simulink model "uavsimblockset_trimModel_Zagi"  (Simulink 8.0)
settings: Solver=ode45  StartTime=0.0  StopTime=10.0  FixedStep=1/30  RelTol=1e-3
undefined symbols (not defined in the file or in its folder): uavsim
libraries: uavsimBlockset_LinearAerodynamicCoefficient x6, uavsimBlockset_LiftCoefficientWithStall x1, aerolibadyn x1, uavsimBlockset_DerivedAerodynamicConditions x1, aerolibtransform2 x1, uavsimBlockset_Environment_calmAtmosphere x1, uavsimBlockset_Quaternion2Rotationvector x1, uavsimblockset_TrimKinematics x1
settings Model: Creator=mstolle  LastModifiedBy=j.bolting
settings DebuggingCC: SolverPrmCheckMsg=none  BusObjectLabelMismatch=error
settings ModelReferenceCC: ModelReferenceMinAlgLoopOccurrences=on

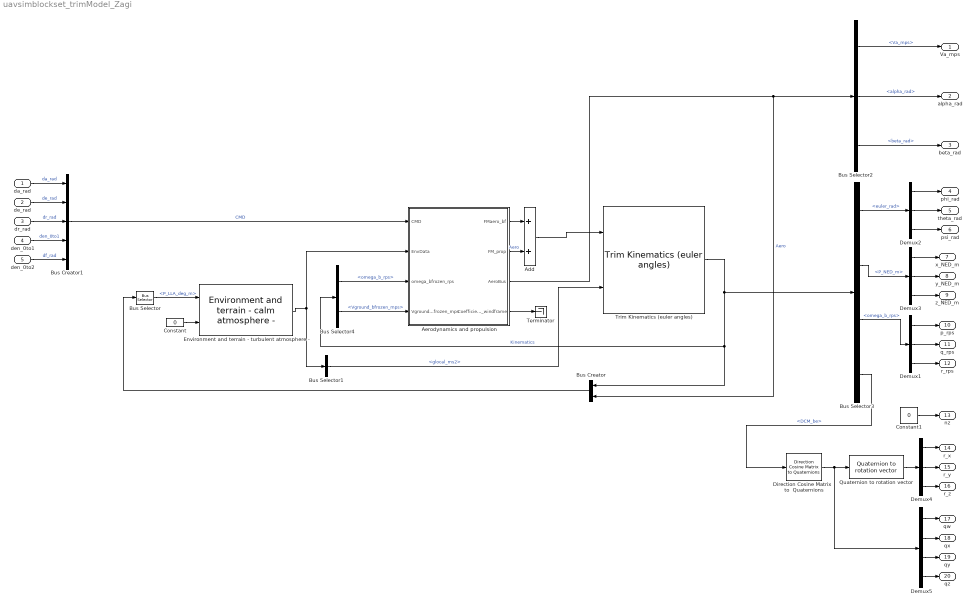
== system uavsimblockset_trimModel_Zagi ==
  da_rad : Inport
  de_rad : Inport  Port=2
  dr_rad : Inport  Port=3
  den_0to1 : Inport  Port=4
  den_0to2 : Inport  Port=5
  Add : Sum
  Aerodynamics and propulsion : Subsystem  AncestorBlock=uavsimBlockset_Zagi_Aerandpropulsion/Zagi aerodynamics and propulsion
      mask Display:
      | port_label('input',1,'CMDBus','texmode','on');
      | port_label('input',2,'EnvDataBus','texmode','on');
      | port_label('input',3,'\omega_{bfrozen,rps}','texmode','on');
      | port_label('input',4,'Vground_{bfrozen,mps}','texmode','on');
      | 
      | port_label('output',1,'FM_{aero}','texmode','on');
      | port_label('output',2,'FM_{propulsion}','texmode','on');
      | port_label('output',3,'AeroBus','texmode','on');
      | port_label('output',4,'C_{wind}','texmode','on');
  Bus Creator1 : BusCreator  Inputs=5  OutDataTypeStr=Bus: CMD  NonVirtualBus=on
  Bus Creator : BusCreator  Inputs=2
  Bus Selector : BusSelector  OutputSignals=Kinematics.Position.P_LLA_deg_m
  Bus Selector1 : BusSelector  OutputSignals=glocal_ms2
  Bus Selector2 : BusSelector  OutputSignals=Va_mps,alpha_rad,beta_rad
  Bus Selector3 : BusSelector  OutputSignals=Attitude.euler_rad,Position.P_NED_m,RotationalVelocity.omega_b_rps,Attitude.DCM_be
  Bus Selector4 : BusSelector  OutputSignals=RotationalVelocity.omega_b_rps,Velocity.Vground_bfrozen_mps
  Constant : Constant  Value=0
  Constant1 : Constant  Value=0
  Demux{1..4} (4 alike) : Demux  Outputs=3
  Demux5 : Demux
  Direction Cosine Matrix   to  Quaternions : aerolibtransform2/Direction Cosine Matrix  to Quaternions
  Environment and terrain - turbulent atmosphere - : uavsimBlockset_Environment_calmAtmosphere/Environment and terrain - calm atmosphere -  SystemSampleTime=-1
  Quaternion to rotation vector : uavsimBlockset_Quaternion2Rotationvector/Quaternion to rotation vector
  Terminator : Terminator
  Trim Kinematics (euler angles) : uavsimblockset_TrimKinematics/Trim Kinematics (euler angles)  mask_inertia=uavsim.zagi.inertiaTensor  mask_mass=uavsim.zagi.mass  mask_P0_ECEF_m=uavsim.mojaveairport_ecef_m  mask_uvw0=[15 0 0]  mask_phithetapsi0=[0 0 0]  mask_omega0=[0 0 0]
  Va_mps : Outport
  alpha_rad : Outport  Port=2
  beta_rad : Outport  Port=3
  phi_rad : Outport  Port=4
  theta_rad : Outport  Port=5
  psi_rad : Outport  Port=6
  x_NED_m : Outport  Port=7
  y_NED_m : Outport  Port=8
  z_NED_m : Outport  Port=9
  p_rps : Outport  Port=10
  q_rps : Outport  Port=11
  r_rps : Outport  Port=12
  nz : Outport  Port=13
  r_x : Outport  Port=14
  r_y : Outport  Port=15
  r_z : Outport  Port=16
  qw : Outport  Port=17
  qx : Outport  Port=18
  qy : Outport  Port=19
  qz : Outport  Port=20
  wires:
  den_0to1/1 -> Bus Creator1/4  "den_0to1"
  de_rad/1 -> Bus Creator1/2  "de_rad"
  da_rad/1 -> Bus Creator1/1  "da_rad"
  dr_rad/1 -> Bus Creator1/3  "dr_rad"
  Bus Creator1/1 -> Aerodynamics and propulsion/1(CMD)  "CMD"
  Environment and terrain - turbulent atmosphere -/1 -> Aerodynamics and propulsion/2(EnvData), Bus Selector1/1
  Bus Selector3/1 -> Demux2/1  "<euler_rad>"
  Demux2/1 -> phi_rad/1
  Demux2/2 -> theta_rad/1
  Demux2/3 -> psi_rad/1
  Bus Selector3/3 -> Demux1/1  "<omega_b_rps>"
  Demux1/1 -> p_rps/1
  Demux1/2 -> q_rps/1
  Demux1/3 -> r_rps/1
  Bus Selector2/1 -> Va_mps/1  "<Va_mps>"
  Bus Selector2/2 -> alpha_rad/1  "<alpha_rad>"
  Bus Selector2/3 -> beta_rad/1  "<beta_rad>"
  Trim Kinematics (euler angles)/1 -> Bus Selector3/1, Bus Creator/1, Bus Selector4/1  "Kinematics"
  Bus Selector4/1 -> Aerodynamics and propulsion/3(omega_bfrozen_rps)  "<omega_b_rps>"
  Bus Selector4/2 -> Aerodynamics and propulsion/4(Vground_bfrozen_mps)  "<Vground_bfrozen_mps>"
  Bus Selector1/1 -> Trim Kinematics (euler angles)/2  "<glocal_ms2>"
  Bus Selector3/2 -> Demux3/1  "<P_NED_m>"
  Demux3/1 -> x_NED_m/1
  Demux3/2 -> y_NED_m/1
  Demux3/3 -> z_NED_m/1
  Constant1/1 -> nz/1
  Bus Selector3/4 -> Direction Cosine Matrix   to  Quaternions/1  "<DCM_be>"
  Direction Cosine Matrix   to  Quaternions/1 -> Demux5/1, Quaternion to rotation vector/1
  Quaternion to rotation vector/1 -> Demux4/1
  Demux4/1 -> r_x/1
  Demux4/2 -> r_y/1
  Demux4/3 -> r_z/1
  Demux5/1 -> qw/1
  Demux5/2 -> qx/1
  Demux5/3 -> qy/1
  Demux5/4 -> qz/1
  den_0to2/1 -> Bus Creator1/5  "df_rad"
  Bus Creator/1 -> Bus Selector/1
  Constant/1 -> Environment and terrain - turbulent atmosphere -/2
  Bus Selector/1 -> Environment and terrain - turbulent atmosphere -/1  "<P_LLA_deg_m>"
  Aerodynamics and propulsion/4(Coefficients_windframe) -> Terminator/1
  Aerodynamics and propulsion/1(FMaero_bf) -> Add/1
  Aerodynamics and propulsion/2(FM_prop) -> Add/2  "Aero"
  Add/1 -> Trim Kinematics (euler angles)/1
  Aerodynamics and propulsion/3(AeroBus) -> Bus Creator/2, Bus Selector2/1  "Aero"

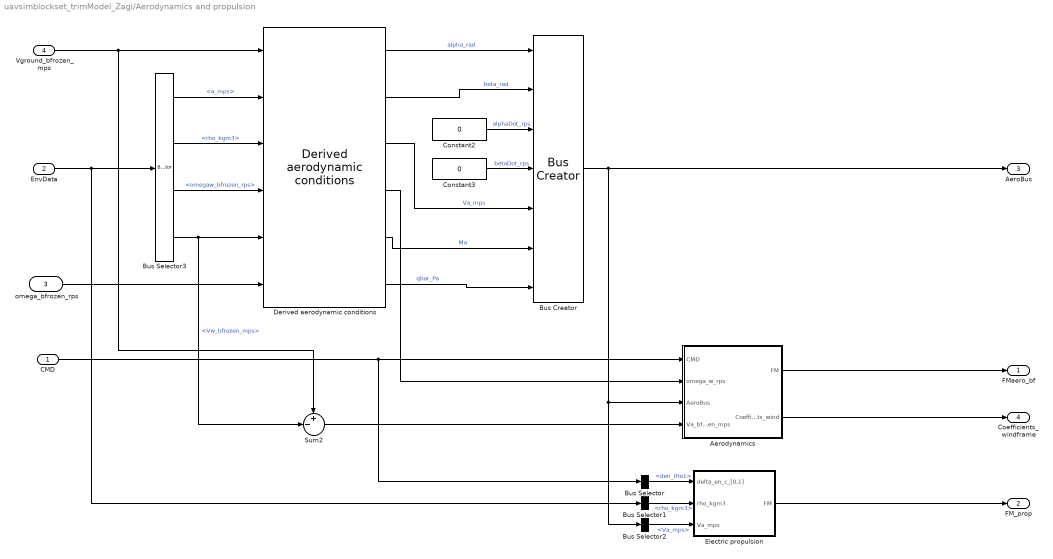
== system uavsimblockset_trimModel_Zagi/Aerodynamics and propulsion ==
  CMD : Inport  OutDataTypeStr=Bus: CMD
  EnvData : Inport  Port=2  OutDataTypeStr=Bus: Environment
  omega_bfrozen_rps : Inport  Port=3
  Vground_bfrozen_mps : Inport  Port=4
  Aerodynamics : Subsystem
  Bus Selector3 : BusSelector  OutputSignals=a_mps,rho_kgm3,omegaw_bfrozen_rps,Vw_bfrozen_mps
  Bus Creator : BusCreator  Inputs=7
  Bus Selector : BusSelector  OutputSignals=den_0to1
  Bus Selector1 : BusSelector  OutputSignals=rho_kgm3
  Bus Selector2 : BusSelector  OutputSignals=Va_mps
  Constant2 : Constant  Value=0
  Constant3 : Constant  Value=0
  Derived aerodynamic conditions : uavsimBlockset_DerivedAerodynamicConditions/Derived aerodynamic conditions
  Electric propulsion : Subsystem  AncestorBlock=uavsimBlockset_ElectricPropulsion/Electric propulsion  mask{mask_C_prop=uavsim.zagi.engine.C_prop, mask_S_prop=uavsim.zagi.engine.S_prop, mask_k_motor=uavsim.zagi.engine.k_motor}
      mask prompts: mask_C_prop "Propeller efficiency constant"; mask_S_prop "Propeller area"; mask_k_motor "Engine constant"
  Sum2 : Sum  Inputs=+-|  SaturateOnIntegerOverflow=on  InputSameDT=on  OutDataTypeStr=Inherit: Same as first input
  FMaero_bf : Outport
  FM_prop : Outport  Port=2
  AeroBus : Outport  Port=3  OutDataTypeStr=Bus: Aero
  Coefficients_windframe : Outport  Port=4
  wires:
  Sum2/1 -> Aerodynamics/4(Va_bfrozen_mps)
  Derived aerodynamic conditions/4 -> Aerodynamics/2(omega_w_rps)
  Bus Creator/1 -> Aerodynamics/3(AeroBus), Bus Selector2/1, AeroBus/1
  Derived aerodynamic conditions/6 -> Bus Creator/7  "qbar_Pa"
  Derived aerodynamic conditions/5 -> Bus Creator/6  "Ma"
  Derived aerodynamic conditions/3 -> Bus Creator/5  "Va_mps"
  Derived aerodynamic conditions/2 -> Bus Creator/2  "beta_rad"
  Derived aerodynamic conditions/1 -> Bus Creator/1  "alpha_rad"
  Vground_bfrozen_mps/1 -> Derived aerodynamic conditions/1, Sum2/1
  Constant3/1 -> Bus Creator/4  "betaDot_rps"
  Constant2/1 -> Bus Creator/3  "alphaDot_rps"
  Bus Selector3/4 -> Sum2/2, Derived aerodynamic conditions/5  "<Vw_bfrozen_mps>"
  Bus Selector3/3 -> Derived aerodynamic conditions/4  "<omegaw_bfrozen_rps>"
  Bus Selector3/2 -> Derived aerodynamic conditions/3  "<rho_kgm3>"
  Bus Selector3/1 -> Derived aerodynamic conditions/2  "<a_mps>"
  Aerodynamics/2(Coefficients_wind) -> Coefficients_windframe/1
  Bus Selector2/1 -> Electric propulsion/3(Va_mps)  "<Va_mps>"
  Bus Selector1/1 -> Electric propulsion/2(rho_kgm3)  "<rho_kgm3>"
  Bus Selector/1 -> Electric propulsion/1(delta_en_c_[0,1])  "<den_0to1>"
  CMD/1 -> Aerodynamics/1(CMD), Bus Selector/1
  Aerodynamics/1(FM) -> FMaero_bf/1
  Electric propulsion/1(FM) -> FM_prop/1
  omega_bfrozen_rps/1 -> Derived aerodynamic conditions/6
  EnvData/1 -> Bus Selector1/1, Bus Selector3/1

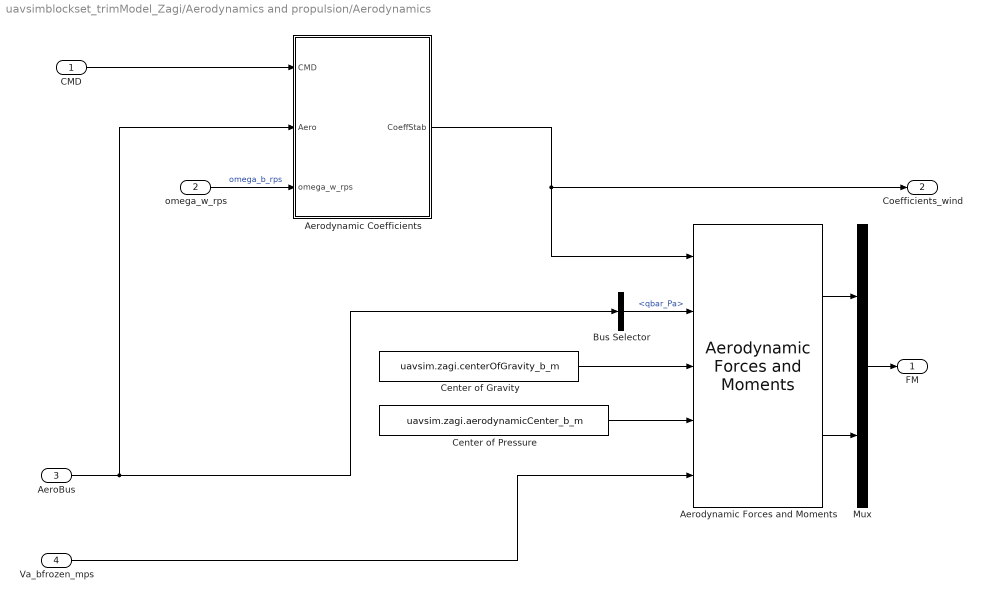
== system uavsimblockset_trimModel_Zagi/Aerodynamics and propulsion/Aerodynamics ==
  CMD : Inport  OutDataTypeStr=Bus: CMD
  omega_w_rps : Inport  Port=2
  AeroBus : Inport  Port=3  OutDataTypeStr=Bus: Aero
  Va_bfrozen_mps : Inport  Port=4
  Aerodynamic Coefficients : Subsystem
  "Aerodynamic Forces and Moments " : aerolibadyn/Aerodynamic Forces and Moments   inputAxes=Wind  outputForceAxes=Body  outputMomentAxes=Body  S=uavsim.zagi.S  b=uavsim.zagi.b  cbar=uavsim.zagi.c
  Bus Selector : BusSelector  OutputSignals=qbar_Pa
  Center of Gravity : Constant  Value=uavsim.zagi.centerOfGravity_b_m  SampleTime=0
  Center of Pressure : Constant  Value=uavsim.zagi.aerodynamicCenter_b_m  SampleTime=0
  Mux : Mux  Inputs=2
  FM : Outport
  Coefficients_wind : Outport  Port=2
  wires:
  Va_bfrozen_mps/1 -> "Aerodynamic Forces and Moments "/5
  omega_w_rps/1 -> Aerodynamic Coefficients/3(omega_w_rps)  "omega_b_rps"
  Bus Selector/1 -> "Aerodynamic Forces and Moments "/2  "<qbar_Pa>"
  Mux/1 -> FM/1
  CMD/1 -> Aerodynamic Coefficients/1(CMD)
  Aerodynamic Coefficients/1(CoeffStab) -> "Aerodynamic Forces and Moments "/1, Coefficients_wind/1
  Center of Pressure/1 -> "Aerodynamic Forces and Moments "/4
  Center of Gravity/1 -> "Aerodynamic Forces and Moments "/3
  "Aerodynamic Forces and Moments "/1 -> Mux/1
  "Aerodynamic Forces and Moments "/2 -> Mux/2
  AeroBus/1 -> Bus Selector/1, Aerodynamic Coefficients/2(Aero)

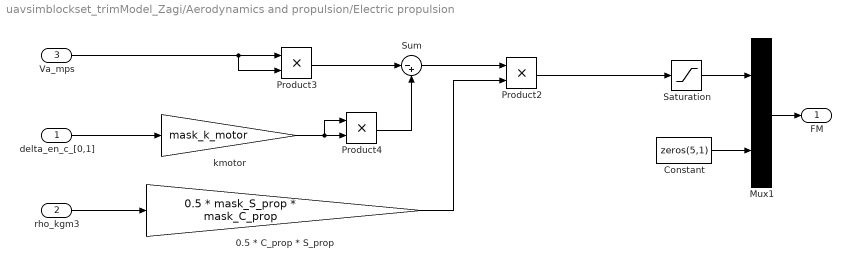
== system uavsimblockset_trimModel_Zagi/Aerodynamics and propulsion/Electric propulsion ==
  delta_en_c_[0,1] : Inport
  rho_kgm3 : Inport  Port=2
  Va_mps : Inport  Port=3
  0.5 * C_prop * S_prop : Gain  Gain=0.5 * mask_S_prop * mask_C_prop
  Constant : Constant  Value=zeros(5,1)
  Mux1 : Mux  Inputs=2
  Product2 : Product  RndMeth=Zero
  Product3 : Product  RndMeth=Zero
  Product4 : Product  RndMeth=Zero
  Saturation : Saturate  UpperLimit=inf  LowerLimit=0
  Sum : Sum  Inputs=|-+
  kmotor : Gain  Gain=mask_k_motor
  FM : Outport
  wires:
  delta_en_c_[0,1]/1 -> kmotor/1
  rho_kgm3/1 -> 0.5 * C_prop * S_prop/1
  Va_mps/1 -> Product3/1, Product3/2
  Product4/1 -> Sum/2
  kmotor/1 -> Product4/2, Product4/1
  0.5 * C_prop * S_prop/1 -> Product2/2
  Product3/1 -> Sum/1
  Sum/1 -> Product2/1
  Product2/1 -> Saturation/1
  Constant/1 -> Mux1/2
  Mux1/1 -> FM/1
  Saturation/1 -> Mux1/1

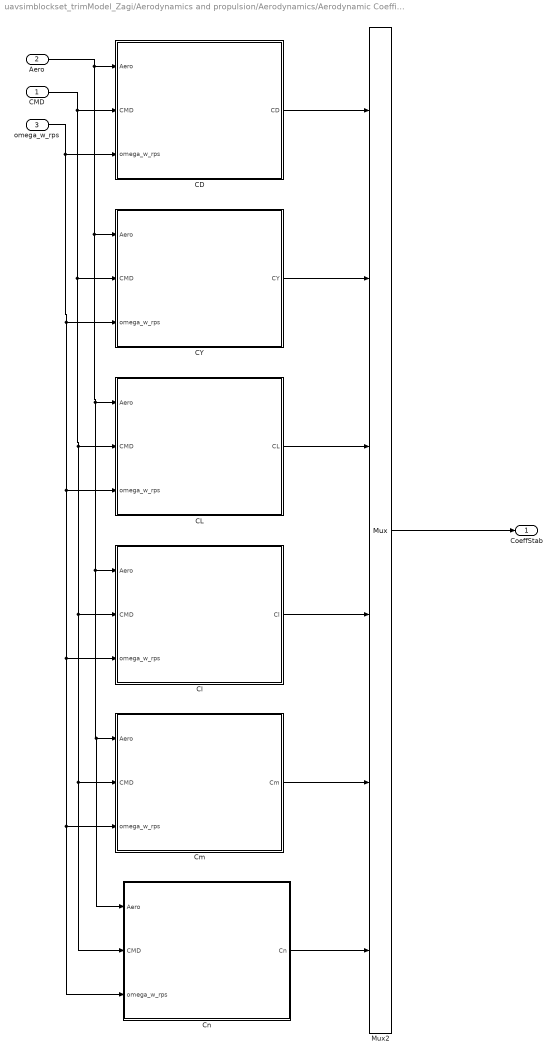
== system uavsimblockset_trimModel_Zagi/Aerodynamics and propulsion/Aerodynamics/Aerodynamic Coefficients ==
  CMD : Inport
  Aero : Inport  Port=2  OutDataTypeStr=Bus: Aero
  omega_w_rps : Inport  Port=3
  CD : Subsystem
  CL : Subsystem
  CY : Subsystem
  Cl : Subsystem
  Cm : Subsystem
  Cn : Subsystem
  Mux2 : Mux  Inputs=6
  CoeffStab : Outport
  wires:
  CY/1(CY) -> Mux2/2
  Cl/1(Cl) -> Mux2/4
  Cn/1(Cn) -> Mux2/6
  Cm/1(Cm) -> Mux2/5
  CD/1(CD) -> Mux2/1
  CL/1(CL) -> Mux2/3
  Aero/1 -> CD/1(Aero), CY/1(Aero), CL/1(Aero), Cl/1(Aero), Cm/1(Aero), Cn/1(Aero)
  CMD/1 -> CD/2(CMD), CY/2(CMD), CL/2(CMD), Cl/2(CMD), Cm/2(CMD), Cn/2(CMD)
  omega_w_rps/1 -> CD/3(omega_w_rps), CY/3(omega_w_rps), CL/3(omega_w_rps), Cl/3(omega_w_rps), Cm/3(omega_w_rps), Cn/3(omega_w_rps)
  Mux2/1 -> CoeffStab/1

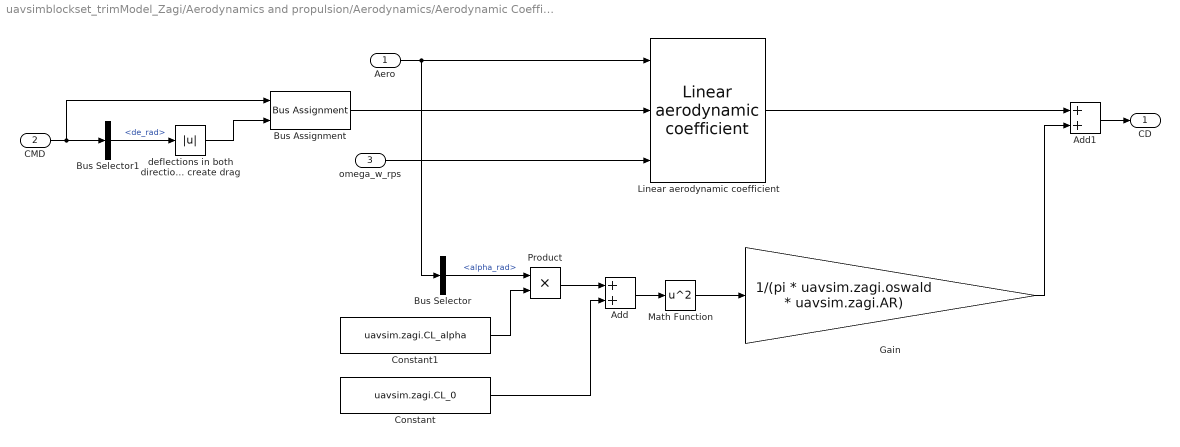
== system uavsimblockset_trimModel_Zagi/Aerodynamics and propulsion/Aerodynamics/Aerodynamic Coefficients/CD ==
  Aero : Inport  OutDataTypeStr=Bus: Aero
  CMD : Inport  Port=2  OutDataTypeStr=Bus: CMD
  omega_w_rps : Inport  Port=3
  Add : Sum
  Add1 : Sum
  Bus Assignment : BusAssignment  AssignedSignals=de_rad
  Bus Selector : BusSelector  OutputSignals=alpha_rad
  Bus Selector1 : BusSelector  OutputSignals=de_rad
  Constant : Constant  Value=uavsim.zagi.CL_0
  Constant1 : Constant  Value=uavsim.zagi.CL_alpha
  Gain : Gain  Gain=1/(pi * uavsim.zagi.oswald * uavsim.zagi.AR)
  Linear aerodynamic coefficient : uavsimBlockset_LinearAerodynamicCoefficient/Linear aerodynamic coefficient  mask_C_0=uavsim.zagi.CD_0  mask_C_alpha=0  mask_C_beta=0  mask_C_alphaDot=0  mask_C_betaDot=0  mask_C_p=0  mask_C_q=0  mask_C_r=0  mask_C_delta_a=0  mask_C_delta_e=uavsim.zagi.CD_de  mask_C_delta_r=0  mask_C_delta_f=0  mask_C_Mach=0
  Math Function : Math  Operator=square  SaturateOnIntegerOverflow=on
  Product : Product  RndMeth=Zero
  deflections in both directions always create drag : Abs
  CD : Outport
  wires:
  Bus Assignment/1 -> Linear aerodynamic coefficient/2
  deflections in both directions always create drag/1 -> Bus Assignment/2
  Bus Selector1/1 -> deflections in both directions always create drag/1  "<de_rad>"
  CMD/1 -> Bus Selector1/1, Bus Assignment/1
  Constant1/1 -> Product/2
  Product/1 -> Add/1
  Bus Selector/1 -> Product/1  "<alpha_rad>"
  omega_w_rps/1 -> Linear aerodynamic coefficient/3
  Aero/1 -> Linear aerodynamic coefficient/1, Bus Selector/1
  Gain/1 -> Add1/2
  Add1/1 -> CD/1
  Linear aerodynamic coefficient/1 -> Add1/1
  Math Function/1 -> Gain/1
  Add/1 -> Math Function/1
  Constant/1 -> Add/2

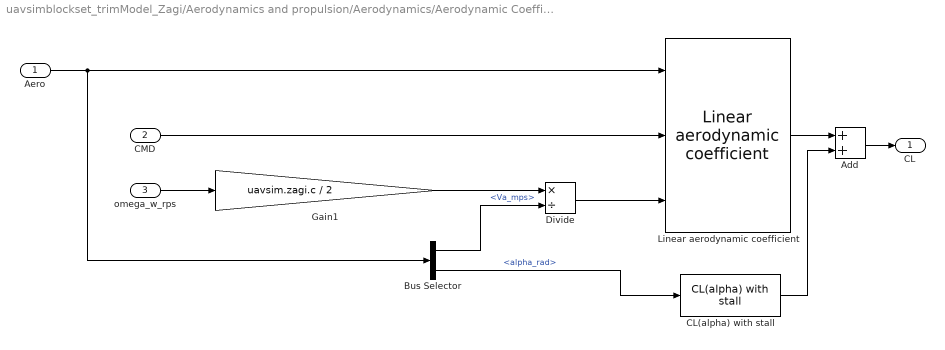
== system uavsimblockset_trimModel_Zagi/Aerodynamics and propulsion/Aerodynamics/Aerodynamic Coefficients/CL ==
  Aero : Inport  OutDataTypeStr=Bus: Aero
  CMD : Inport  Port=2  OutDataTypeStr=Bus: CMD
  omega_w_rps : Inport  Port=3
  Add : Sum
  Bus Selector : BusSelector  OutputSignals=Va_mps,alpha_rad
  CL(alpha) with stall : uavsimBlockset_LiftCoefficientWithStall/CL(alpha) with stall  mask_M=uavsim.zagi.stall.M  mask_alpha0=uavsim.zagi.alpha0  mask_CL_0=uavsim.zagi.CL_0  mask_CL_alpha=uavsim.zagi.CL_alpha
  Divide : Product  Inputs=*/
  Gain1 : Gain  Gain=uavsim.zagi.c / 2
  Linear aerodynamic coefficient : uavsimBlockset_LinearAerodynamicCoefficient/Linear aerodynamic coefficient  mask_C_0=0  mask_C_alpha=0  mask_C_beta=0  mask_C_alphaDot=0  mask_C_betaDot=0  mask_C_p=0  mask_C_q=uavsim.zagi.CL_q  mask_C_r=0  mask_C_delta_a=0  mask_C_delta_e=uavsim.zagi.CL_de  mask_C_delta_r=0  mask_C_delta_f=0  mask_C_Mach=0
  CL : Outport
  wires:
  Add/1 -> CL/1
  CL(alpha) with stall/1 -> Add/2
  Bus Selector/2 -> CL(alpha) with stall/1  "<alpha_rad>"
  Aero/1 -> Bus Selector/1, Linear aerodynamic coefficient/1
  omega_w_rps/1 -> Gain1/1
  CMD/1 -> Linear aerodynamic coefficient/2
  Gain1/1 -> Divide/1
  Bus Selector/1 -> Divide/2  "<Va_mps>"
  Divide/1 -> Linear aerodynamic coefficient/3
  Linear aerodynamic coefficient/1 -> Add/1

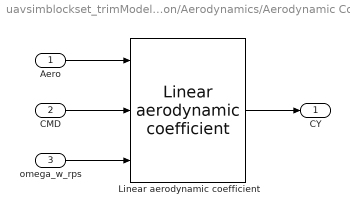
== system uavsimblockset_trimModel_Zagi/Aerodynamics and propulsion/Aerodynamics/Aerodynamic Coefficients/CY ==
  Aero : Inport  OutDataTypeStr=Bus: Aero
  CMD : Inport  Port=2  OutDataTypeStr=Bus: CMD
  omega_w_rps : Inport  Port=3
  Linear aerodynamic coefficient : uavsimBlockset_LinearAerodynamicCoefficient/Linear aerodynamic coefficient  mask_C_0=0  mask_C_alpha=0  mask_C_beta=uavsim.zagi.CY_beta  mask_C_alphaDot=0  mask_C_betaDot=0  mask_C_p=0  mask_C_q=0  mask_C_r=0  mask_C_delta_a=0  mask_C_delta_e=0  mask_C_delta_r=0  mask_C_delta_f=0  mask_C_Mach=0
  CY : Outport
  wires:
  omega_w_rps/1 -> Linear aerodynamic coefficient/3
  Linear aerodynamic coefficient/1 -> CY/1
  Aero/1 -> Linear aerodynamic coefficient/1
  CMD/1 -> Linear aerodynamic coefficient/2

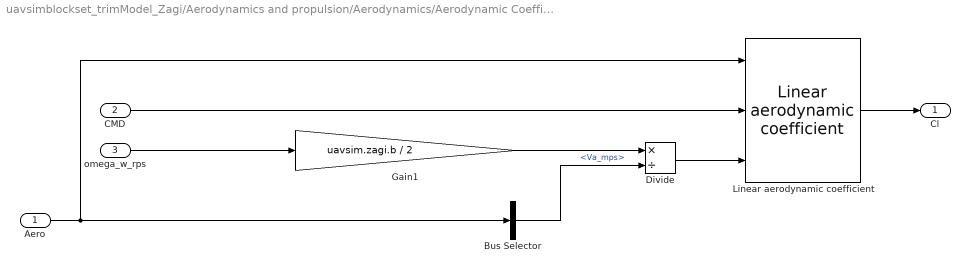
== system uavsimblockset_trimModel_Zagi/Aerodynamics and propulsion/Aerodynamics/Aerodynamic Coefficients/Cl ==
  Aero : Inport  OutDataTypeStr=Bus: Aero
  CMD : Inport  Port=2  OutDataTypeStr=Bus: CMD
  omega_w_rps : Inport  Port=3
  Bus Selector : BusSelector  OutputSignals=Va_mps
  Divide : Product  Inputs=*/
  Gain1 : Gain  Gain=uavsim.zagi.b / 2
  Linear aerodynamic coefficient : uavsimBlockset_LinearAerodynamicCoefficient/Linear aerodynamic coefficient  mask_C_0=0  mask_C_alpha=0  mask_C_beta=uavsim.zagi.Cl_beta  mask_C_alphaDot=0  mask_C_betaDot=0  mask_C_p=uavsim.zagi.Cl_p  mask_C_q=0  mask_C_r=uavsim.zagi.Cl_r  mask_C_delta_a=uavsim.zagi.Cl_da  mask_C_delta_e=0  mask_C_delta_r=0  mask_C_delta_f=0  mask_C_Mach=0
  Cl : Outport
  wires:
  Linear aerodynamic coefficient/1 -> Cl/1
  Divide/1 -> Linear aerodynamic coefficient/3
  Bus Selector/1 -> Divide/2  "<Va_mps>"
  Gain1/1 -> Divide/1
  CMD/1 -> Linear aerodynamic coefficient/2
  omega_w_rps/1 -> Gain1/1
  Aero/1 -> Linear aerodynamic coefficient/1, Bus Selector/1

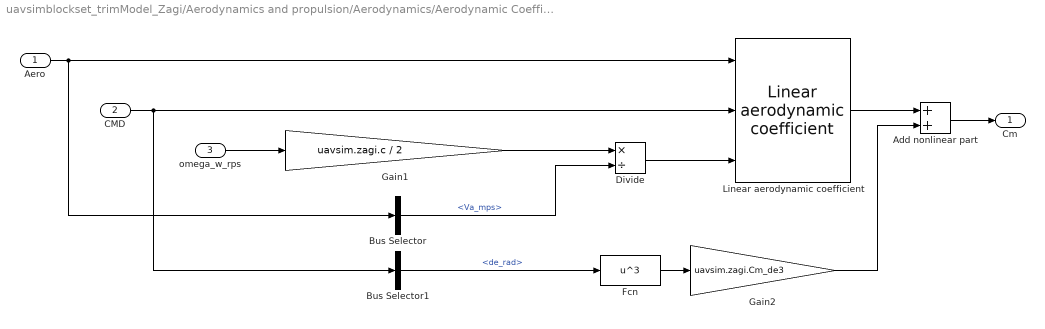
== system uavsimblockset_trimModel_Zagi/Aerodynamics and propulsion/Aerodynamics/Aerodynamic Coefficients/Cm ==
  Aero : Inport  OutDataTypeStr=Bus: Aero
  CMD : Inport  Port=2  OutDataTypeStr=Bus: CMD
  omega_w_rps : Inport  Port=3
  Add nonlinear part : Sum
  Bus Selector : BusSelector  OutputSignals=Va_mps
  Bus Selector1 : BusSelector  OutputSignals=de_rad
  Divide : Product  Inputs=*/
  Fcn : Fcn  Expr=u^3
  Gain1 : Gain  Gain=uavsim.zagi.c / 2
  Gain2 : Gain  Gain=uavsim.zagi.Cm_de3
  Linear aerodynamic coefficient : uavsimBlockset_LinearAerodynamicCoefficient/Linear aerodynamic coefficient  mask_C_0=uavsim.zagi.Cm_0  mask_C_alpha=uavsim.zagi.Cm_alpha  mask_C_beta=0  mask_C_alphaDot=0  mask_C_betaDot=0  mask_C_p=0  mask_C_q=uavsim.zagi.Cm_q  mask_C_r=0  mask_C_delta_a=0  mask_C_delta_e=uavsim.zagi.Cm_de  mask_C_delta_r=0  mask_C_delta_f=0  mask_C_Mach=0
  Cm : Outport
  wires:
  Bus Selector1/1 -> Fcn/1  "<de_rad>"
  Gain2/1 -> Add nonlinear part/2
  Fcn/1 -> Gain2/1
  Add nonlinear part/1 -> Cm/1
  Linear aerodynamic coefficient/1 -> Add nonlinear part/1
  Divide/1 -> Linear aerodynamic coefficient/3
  Bus Selector/1 -> Divide/2  "<Va_mps>"
  Gain1/1 -> Divide/1
  CMD/1 -> Bus Selector1/1, Linear aerodynamic coefficient/2
  omega_w_rps/1 -> Gain1/1
  Aero/1 -> Bus Selector/1, Linear aerodynamic coefficient/1

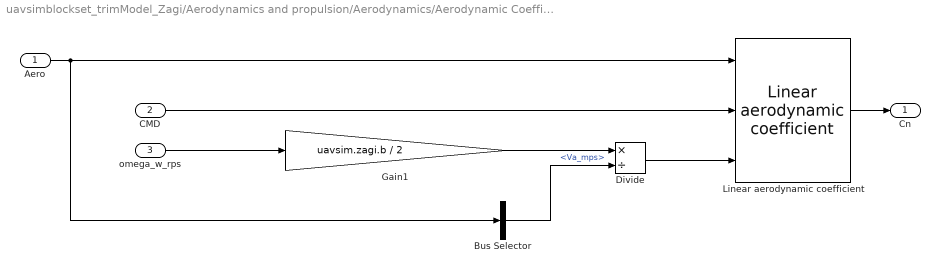
== system uavsimblockset_trimModel_Zagi/Aerodynamics and propulsion/Aerodynamics/Aerodynamic Coefficients/Cn ==
  Aero : Inport  OutDataTypeStr=Bus: Aero
  CMD : Inport  Port=2  OutDataTypeStr=Bus: CMD
  omega_w_rps : Inport  Port=3
  Bus Selector : BusSelector  OutputSignals=Va_mps
  Divide : Product  Inputs=*/
  Gain1 : Gain  Gain=uavsim.zagi.b / 2
  Linear aerodynamic coefficient : uavsimBlockset_LinearAerodynamicCoefficient/Linear aerodynamic coefficient  mask_C_0=0  mask_C_alpha=0  mask_C_beta=uavsim.zagi.Cn_beta  mask_C_alphaDot=0  mask_C_betaDot=0  mask_C_p=uavsim.zagi.Cn_p  mask_C_q=0  mask_C_r=uavsim.zagi.Cn_r  mask_C_delta_a=uavsim.zagi.Cn_da  mask_C_delta_e=0  mask_C_delta_r=0  mask_C_delta_f=0  mask_C_Mach=0
  Cn : Outport
  wires:
  Aero/1 -> Linear aerodynamic coefficient/1, Bus Selector/1
  omega_w_rps/1 -> Gain1/1
  CMD/1 -> Linear aerodynamic coefficient/2
  Gain1/1 -> Divide/1
  Bus Selector/1 -> Divide/2  "<Va_mps>"
  Divide/1 -> Linear aerodynamic coefficient/3
  Linear aerodynamic coefficient/1 -> Cn/1
